simulink model "Task_1A"  (R2022a)
settings: Solver=VariableStepAuto  StartTime=0.0  StopTime=10.0  RelTol=1e-3
values from neighbouring files (symbols this model uses):
  K = 1    [Parameter_Setup.m]
  La = 0.001    [Parameter_Setup.m]
  N = 1    [Parameter_Setup.m]
  Ra = 1    [Parameter_Setup.m]
libraries: simulink x2
settings Model: Creator=jpcas  LastModifiedBy=jpcas

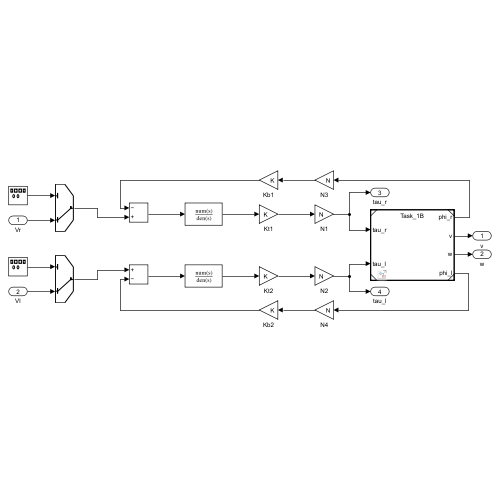
[thumbnail: Simulink's stored preview of the top-level diagram]
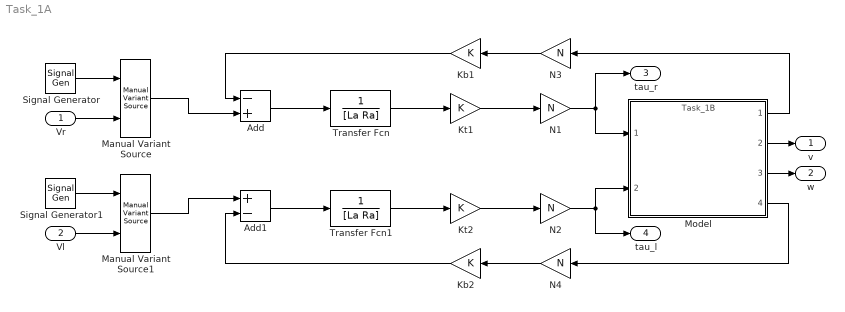
== system Task_1A ==
  Vr : Inport
  Vl : Inport  Port=2
  Add : Sum  Inputs=-+
  Add1 : Sum  Inputs=+-
  Kb1 : Gain  Gain=K
  Kb2 : Gain  Gain=K
  Kt1 : Gain  Gain=K
  Kt2 : Gain  Gain=K
  Manual Variant Source : simulink/Signal Routing/Manual Variant Source  NumChoices=2  LabelModeActiveChoice=V_2
  Manual Variant Source1 : simulink/Signal Routing/Manual Variant Source  NumChoices=2  LabelModeActiveChoice=V_2
  Model : ModelReference  ModelNameDialog=Task_1B.slx  SimulationMode=Normal  ModelReferenceVersion=1.16
  N{1..4} (4 alike) : Gain  Gain=N
  Signal Generator : SignalGenerator  Units=rad/sec
  Signal Generator1 : SignalGenerator  Units=rad/sec
  Transfer Fcn : TransferFcn  Denominator=[La Ra]
  Transfer Fcn1 : TransferFcn  Denominator=[La Ra]
  v : Outport
  w : Outport  Port=2
  tau_r : Outport  Port=3
  tau_l : Outport  Port=4
  wires:
  N1/1 -> tau_r/1, Model/1
  Transfer Fcn/1 -> Kt1/1
  Kt1/1 -> N1/1
  Transfer Fcn1/1 -> Kt2/1
  Kt2/1 -> N2/1
  N2/1 -> tau_l/1, Model/2
  Add/1 -> Transfer Fcn/1
  Add1/1 -> Transfer Fcn1/1
  Model/4 -> N4/1
  Model/1 -> N3/1
  N4/1 -> Kb2/1
  N3/1 -> Kb1/1
  Kb1/1 -> Add/1
  Kb2/1 -> Add1/2
  Manual Variant Source1/1 -> Add1/1
  Manual Variant Source/1 -> Add/2
  Signal Generator/1 -> Manual Variant Source/1
  Signal Generator1/1 -> Manual Variant Source1/1
  Vr/1 -> Manual Variant Source/2
  Vl/1 -> Manual Variant Source1/2
  Model/3 -> w/1
  Model/2 -> v/1
